simulink model "PVArray"  (R2016a)
settings: Solver=ode45  StartTime=0.0  StopTime=100  RelTol=1e-3
values from neighbouring files (symbols this model uses):
  Io = (Isc - (Voc - Rs*Isc)/ Rsh) * exp(-Voc/ (m*Vt))    [SolarPanelModel.m]
  Is = Io * exp(Voc/ (m*Vt)) + Voc/ Rsh    [SolarPanelModel.m]
  m = sol(1)    [SolarPanelModel.m]
  Rs = sol(3)    [SolarPanelModel.m]
  Rsh = sol(2)    [SolarPanelModel.m]
  Vt = K*Tc/ q    (= 0.0291654375)    [SolarPanelModel.m]
libraries: powerlib x7, spsPVarrayModel x1, re_lib x1
settings Model: Creator=frede  LastModifiedBy=frede
settings DataIOCC: LimitDataPoints=on  SaveFormat=Array
settings HardwareCC: ProdBitPerPointer=32  ProdLargestAtomicFloat=None  ProdIntDivRoundTo=Undefined  ProdEndianess=Unspecified  ProdWordSize=32  ProdHWDeviceType=32-bit Generic
settings ModelReferenceCC: PropagateSignalLabelsOutOfModel=off
settings ConfigComp: CovModelRefEnable=Off

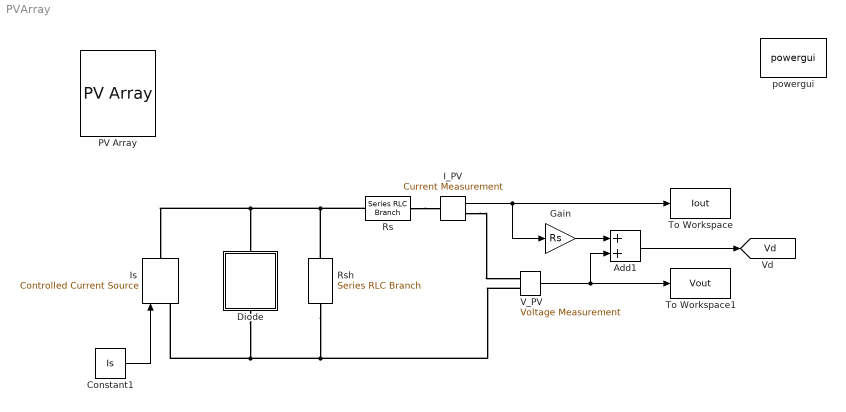
== system PVArray ==
  Add1 : Sum
  Constant1 : Constant  Value=Is
  Diode : Subsystem  AncestorBlock=re_lib/Solar/PV Array/Diode Rsh
      mask Display:
      | plot(-75,-50,100,150, [-15 -15 43 -15 -15 -75],[50 8 50 92 50 50], ...
      |     [43 43],[8 94],[100 43], [50 50])
  Gain : Gain  Gain=Rs
  I_PV : powerlib/Measurements/Current Measurement  PhasorSimulation=off  OutputType=Complex  PSBequivalent=0
  Is : powerlib/Electrical Sources/Controlled Current Source  Initialize=on  Source_Type=DC  Amplitude=Is  Phase=0  Frequency=0  Measurements=None
  PV Array : re_lib/Solar/PV Array  Npar=40  Nser=10  PlotType=array @ 1000 W/m2 & specified temperatures  S_vec="[ 1000  500  100 ]"  Temp_C_vec="[ 45 25  ]"  ModuleName=1Soltech 1STH-215-P  PlotWhenSelected=off  Pm=213.15  Ncell=60  Voc=36.3  Isc=7.84  Vm=29  Im=7.35  beta_Voc_pc=-0.36099  alpha_Isc_pc=0.102  beta_Voc=-0.13104  alpha_Isc=0.007997  IL=7.8649  I0=2.9259e-10  nI=0.98117  Rsh=313.3991  Rs=0.39383  BAL=off  Tc=1e-6  Tfilter=5e-5
  Rs : powerlib/Elements/Series RLC Branch  LConnTagsString=__new0  RConnTagsString=__new0  BranchType=R  Resistance=Rs  Inductance=1e-3  SetiL0=off  InitialCurrent=0  Capacitance=1e-6  Setx0=off  InitialVoltage=0  Measurements=None
  Rsh : powerlib/Elements/Series RLC Branch  LConnTagsString=__new0  RConnTagsString=__new0  BranchType=R  Resistance=Rsh  Inductance=1e-3  SetiL0=off  InitialCurrent=0  Capacitance=1e-6  Setx0=off  InitialVoltage=0  Measurements=None
  To Workspace : ToWorkspace  VariableName=Iout  SampleTime=-1
  To Workspace1 : ToWorkspace  VariableName=Vout  SampleTime=-1
  V_PV : powerlib/Measurements/Voltage Measurement  PhasorSimulation=off  OutputType=Complex  PSBequivalent=0
  powergui : powerlib/powergui  Priority=1  SimulationMode=Continuous  SolverType=Tustin/Backward Euler (TBE)  SampleTime=50e-6  frequency=60  SPID=off  DisableSnubberDevices=off  DisableRonSwitches=off  DisableVfSwitches=off  SwTol=0  DisplayEquations=off  Interpol=off  ExternalGateDelay=off  methode=off  Ts=10  FunctionMessages=off  echomessages=off  HookPort=off  EnableUseOfTLC=off  x0status=blocks  frequencyindice=0  Pbase=100e6  ErrMax=1e-4  Iterations=50  UnitsV=kV  UnitsW=MW  buscounter=0  RestoreLinks=warning  ResistiveCurrentMeasurement=off  Frange=[0:2:500]  Ylog=off  Xlog=on  ShowGrid=off  save=off  variable=ZData  structure=0  ZoomFFT=off  StartTime=0.0  cycles=1  DisplayStyle=1  fundamental=60  FreqAxis=off  MaxFrequency=1000  frequencyindicesteady=1  RmsSteady=1  display=off
  tag scope: Vd=global
  wires:
  V_PV/1 -> Add1/2, To Workspace1/1
  Constant1/1 -> Is/1
  I_PV/1 -> To Workspace/1, Gain/1
  Gain/1 -> Add1/1
  Add1/1 -> [Vd]
  connections:
  V_PV/LConn2 -- Rsh/RConn1 -- Is/LConn1 -- Diode/RConn1
  Rs/LConn1 -- Rsh/LConn1 -- Is/RConn1 -- Diode/LConn1
  I_PV/RConn1 -- V_PV/LConn1
  Rs/RConn1 -- I_PV/LConn1

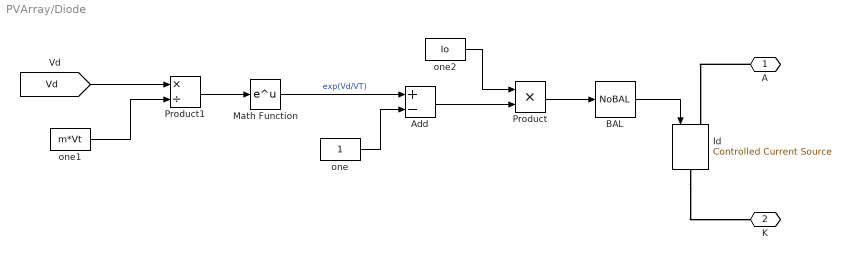
== system PVArray/Diode ==
  Add : Sum  Inputs=+-
  BAL : spsPVarrayModel/NoBAL  VariantControl=NoBAL
  Id : powerlib/Electrical Sources/Controlled Current Source  Initialize=on  Source_Type=AC  Amplitude=0  Phase=0  Frequency=0  Measurements=None
  Math Function : Math  SaturateOnIntegerOverflow=on
  Product : Product  RndMeth=Zero
  Product1 : Product  Inputs=*/  RndMeth=Zero
  one : Constant
  one1 : Constant  Value=m*Vt
  one2 : Constant  Value=Io
  A : PMIOPort  Port=1  Side=Left
  K : PMIOPort  Port=2  Side=Right
  wires:
  BAL/1 -> Id/1
  Math Function/1 -> Add/1  "exp(Vd/VT)"
  Product/1 -> BAL/1
  Product1/1 -> Math Function/1
  one/1 -> Add/2
  Add/1 -> Product/2
  one2/1 -> Product/1
  [Vd] -> Product1/1
  one1/1 -> Product1/2
  connections:
  Id/RConn1 -- K/RConn1
  A/RConn1 -- Id/LConn1
